simulink model "SatelliteModel"  (R2014b)
settings: Solver=ode45  StartTime=0.0  StopTime=10.0  RelTol=1e-3
undefined symbols (not defined in the file or in its folder): NAVtable1, PRNtable
libraries: dspswit3 x3, simulink x2, commsynccomp2 x2
settings Model: Creator=Alexandre Buscher  LastModifiedBy=Alexandre Buscher

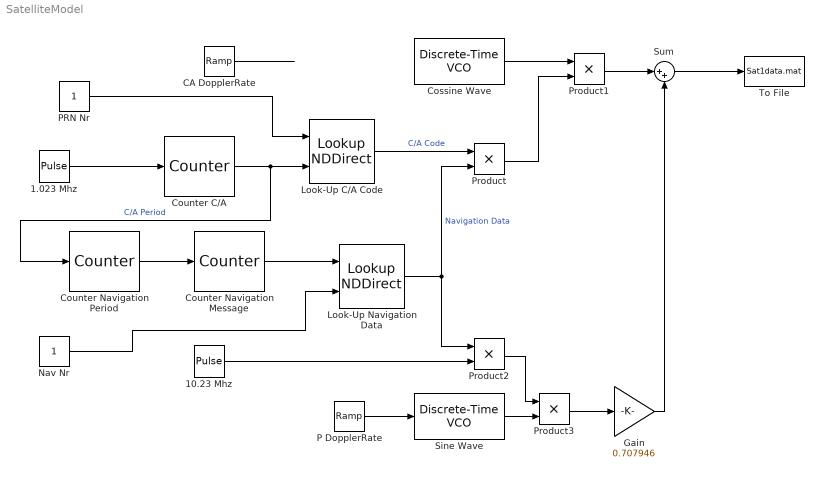
== system SatelliteModel ==
  "1.023 Mhz " : DiscretePulseGenerator  PulseType=Time based  Period=1/1023000  PulseWidth=50
  10.23 Mhz : DiscretePulseGenerator  PulseType=Time based  Period=1/10230000  PulseWidth=50
  CA DopplerRate : simulink/Sources/Ramp  slope=1  start=0  X0=0  VectorParams1D=off
  "Cossine Wave " : commsynccomp2/Discrete-Time VCO  Ac=1  Fc=1227600000  Kc=0.2  Ph=0  ts=1/12000000
  Counter Navigation Message : dspswit3/Counter  Direction=Up  CountEvent=Falling edge  CounterSize=User defined  MaxCount=1500  InitialCount=0  Output=Count  HitValue=32  ResetInput=off  SamplesPerFrame=1  Ts=1  CntDtype=double  HitDtype=Logical
  Counter Navigation Period : dspswit3/Counter  Direction=Up  CountEvent=Falling edge  CounterSize=User defined  MaxCount=20  InitialCount=0  Output=Count  HitValue=32  ResetInput=off  SamplesPerFrame=1  Ts=1  CntDtype=double  HitDtype=Logical
  Counter C/A : dspswit3/Counter  Direction=Up  CountEvent=Falling edge  CounterSize=User defined  MaxCount=1022  InitialCount=0  Output=Count  HitValue=32  ResetInput=off  SamplesPerFrame=1  Ts=1  CntDtype=double  HitDtype=Logical
  Gain : Gain  Gain=0.707946
  Look-Up C/A Code : LookupNDDirect  Table=PRNtable
  Look-Up Navigation Data : LookupNDDirect  Table=NAVtable1
  Nav Nr : Constant  OutMin=1  OutMax=16
  P DopplerRate : simulink/Sources/Ramp  slope=1  start=0  X0=0
  PRN Nr : Constant  OutMin=1  OutMax=32
  Product{,1..3} (4 alike) : Product
  Sine Wave : commsynccomp2/Discrete-Time VCO  Ac=1  Fc=1575420000  Kc=1  Ph=pi/2  ts=1/12000000
  Sum : Sum  Inputs=|++
  To File : ToFile  Filename=Sat1data.mat  MatrixName=Sat1data  SaveFormat=Timeseries
  wires:
  "1.023 Mhz "/1 -> Counter C/A/1
  Counter C/A/1 -> Counter Navigation Period/1, Look-Up C/A Code/2  "C/A Period"
  PRN Nr/1 -> Look-Up C/A Code/1
  Look-Up C/A Code/1 -> Product/1  "C/A Code"
  "Cossine Wave "/1 -> Product1/1
  Product/1 -> Product1/2
  Counter Navigation Period/1 -> Counter Navigation Message/1
  Look-Up Navigation Data/1 -> Product2/1, Product/2  "Navigation Data"
  Counter Navigation Message/1 -> Look-Up Navigation Data/1
  10.23 Mhz/1 -> Product2/2
  P DopplerRate/1 -> Sine Wave/1
  Sine Wave/1 -> Product3/2
  Product2/1 -> Product3/1
  Product3/1 -> Gain/1
  Gain/1 -> Sum/2
  Product1/1 -> Sum/1
  Sum/1 -> To File/1
  Nav Nr/1 -> Look-Up Navigation Data/2
  CA DopplerRate/1 -> ?
  ? -> "Cossine Wave "/1
